simulink model "HIL_simu"  (R2019b)
settings: Solver=VariableStepAuto  StartTime=0.0  StopTime=10.0  RelTol=1e-3
values from neighbouring files (symbols this model uses):
  B = 0.003    [HIL.m]
  b = 7.2e-5    (= 7.2e-05)    [HIL.m]    (also in SIL.m = 4.2697318139e-06)
  C_r = u*Kc/R    (= 0.0265986622074)    [HIL.m]
  Jeq = 0.029*l^2 + J    (= 0.0002543)    [HIL.m]
  K1 = 0.007    [HIL.m]
  K2 = 1    [HIL.m]
  Kc = Ke    (= 0.0241)    [HIL.m]    (also in SIL.m)
  Ke = 24.1e-3    (= 0.0241)    [HIL.m]    (also in SIL.m = 0.024114385317)
  L = 0.42e-3    (= 0.00042)    [HIL.m]    (also in SIL.m)
  R = 2.99    [HIL.m]    (also in SIL.m)
libraries: simulink_extras x2, simulink x1
settings Model: Creator=tclaverie303  LastModifiedBy=tclaverie303

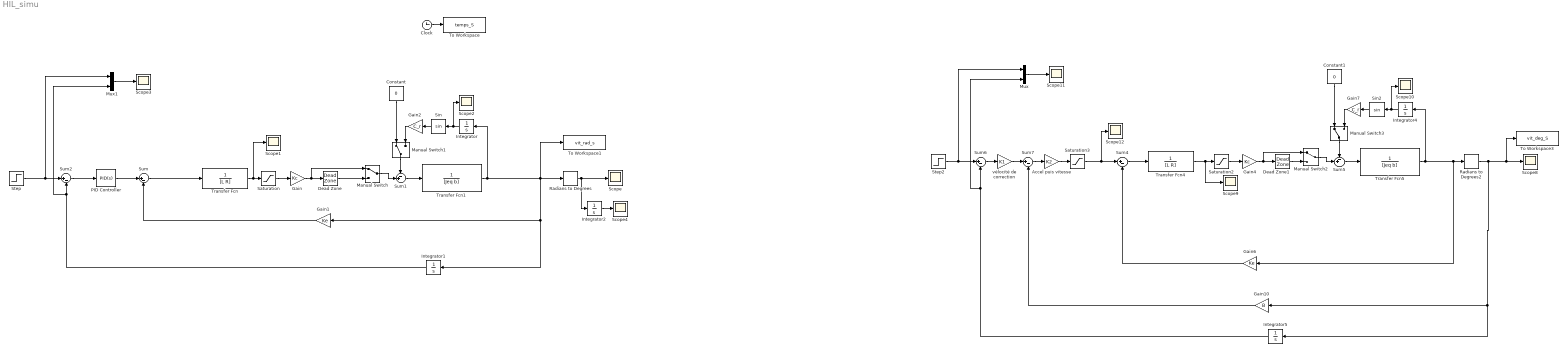
== system HIL_simu ==
  Accel puis vitesse : Gain  Gain=K2
  Clock : Clock
  Constant : Constant  Value=0
  Constant1 : Constant  Value=0
  Dead Zone : DeadZone  SaturateOnIntegerOverflow=on
  Dead Zone1 : DeadZone  SaturateOnIntegerOverflow=on
  Gain : Gain  Gain=Kc
  Gain1 : Gain  Gain=Ke
  Gain10 : Gain  Gain=B
  Gain2 : Gain  Gain=C_r
  Gain4 : Gain  Gain=Kc
  Gain6 : Gain  Gain=Ke
  Gain7 : Gain  Gain=C_r
  Integrator{,1..2,4..5} (5 alike) : Integrator
  Manual Switch{,1..3} (4 alike) : ManualSwitch
  Mux : Mux  Inputs=2
  Mux1 : Mux  Inputs=2
  PID Controller : simulink/Continuous/PID Controller  Controller=PID  Form=Parallel  TimeDomain=Continuous-time  SampleTime=-1  IntegratorMethod=Forward Euler  FilterMethod=Forward Euler  ControllerParametersSource=internal  P=1.5  I=0  D=0.5  UseFilter=on  N=4000  TunerSelectOption=Transfer Function Based (PID Tuner App)  InitialConditionSource=internal  InitialConditionForIntegrator=0  InitialConditionForFilter=0  DifferentiatorICPrevScaledInput=0  ExternalReset=none  TrackingMode=off  Kt=1  LimitOutput=off  UpperSaturationLimit=inf  LowerSaturationLimit=-inf  LinearizeAsGain=on  AntiWindupMode=none  Kb=1  POutMin=[]  POutMax=[]  IOutMin=[]  IOutMax=[]  DOutMin=[]  DOutMax=[]  NOutMin=[]  NOutMax=[]  SumOutMin=[]  SumOutMax=[]  SaturationOutMin=[]  SaturationOutMax=[]  PParamMin=[]  PParamMax=[]  IParamMin=[]  IParamMax=[]  DParamMin=[]  DParamMax=[]  NParamMin=[]  NParamMax=[]  KbParamMin=[]  KbParamMax=[]  KtParamMin=[]  KtParamMax=[]  KbOutMin=[]  KbOutMax=[]  KtOutMin=[]  KtOutMax=[]  IntegratorOutMin=[]  IntegratorOutMax=[]  FilterOutMin=[]  FilterOutMax=[]  SumI1OutMin=[]  SumI1OutMax=[]  SumI2OutMin=[]  SumI2OutMax=[]  SumI3OutMin=[]  SumI3OutMax=[]  SumI4OutMin=[]  SumI4OutMax=[]  SumDOutMin=[]  SumDOutMax=[]  DifferentiatorOutMin=[]  DifferentiatorOutMax=[]  FilterDiffOutCoefMin=[]  FilterDiffOutCoefMax=[]  ReciprocalOutMin=[]  ReciprocalOutMax=[]  SumDenOutMin=[]  SumDenOutMax=[]  SumNumOutMin=[]  SumNumOutMax=[]  DivideOutMin=[]  DivideOutMax=[]  IntegratorContinuousStateAttributes=''  IntegratorStateMustResolveToSignalObject=off  IntegratorRTWStateStorageClass=Auto  FilterContinuousStateAttributes=''  FilterStateMustResolveToSignalObject=off  FilterRTWStateStorageClass=Auto  ParallelPVariant=InternalParameters  IdealPVariant=Disabled  IVariant=InternalParameters  DVariant=InternalParameters  IntegratorVariant=Continuous  SatVariant=Disabled  AWVariant=Passthrough  PCopyVariant=Disabled  TRVariant=Disabled  FdbkBlocksVariant=Forward  IdealPFdbkVariant=Disabled  SatFdbkVariant=Disabled  DerivativeFilterVariant=ContFilter  NVariant=InternalParameters  NCopyVariant=Disabled  FilterICVariant=InternalICsFilter  IntegratorICVariant=InternalICs  ExternalResetVariant=Disabled  TRSumVariant=Passthrough  SumFdbkVariant=Disabled  SumVariant=Sum_PID
  Radians to Degrees : simulink_extras/Transformations/Radians to Degrees
  Radians to Degrees2 : simulink_extras/Transformations/Radians to Degrees
  Saturation : Saturate
  Saturation2 : Saturate
  Saturation3 : Saturate
  Scope{,1..4,8..12} (10 alike) : Scope
  Sin : Trigonometry
  Sin2 : Trigonometry
  Step : Step  After=3.3  SampleTime=0
  Step2 : Step  After=3.3  SampleTime=0
  Sum{,2,4,6..7} (5 alike) : Sum  Inputs=|+-
  Sum1 : Sum  Inputs=-+|
  Sum5 : Sum  Inputs=-+|
  To Workspace : ToWorkspace  VariableName=temps_S  SaveFormat=Timeseries  SampleTime=-1
  To Workspace1 : ToWorkspace  VariableName=vit_rad_s  SaveFormat=Timeseries  SampleTime=-1
  To Workspace3 : ToWorkspace  VariableName=vit_deg_S  SaveFormat=Timeseries  SampleTime=-1
  Transfer Fcn : TransferFcn  Denominator=[L R]
  Transfer Fcn1 : TransferFcn  Denominator=[Jeq b]
  Transfer Fcn4 : TransferFcn  Denominator=[L R]
  Transfer Fcn5 : TransferFcn  Denominator=[Jeq b]
  "vélocité de correction " : Gain  Gain=K1
  wires:
  Sum/1 -> Transfer Fcn/1
  Transfer Fcn/1 -> Scope1/1, Saturation/1
  Saturation/1 -> Gain/1
  Clock/1 -> To Workspace/1
  Gain1/1 -> Sum/2
  Sum1/1 -> Transfer Fcn1/1
  Integrator/1 -> Scope2/1, Sin/1
  Sin/1 -> Gain2/1
  Radians to Degrees/1 -> Integrator2/1, Scope/1
  Gain/1 -> Manual Switch/1, Dead Zone/1
  Dead Zone/1 -> Manual Switch/2
  Manual Switch/1 -> Sum1/2
  Gain2/1 -> Manual Switch1/2
  Manual Switch1/1 -> Sum1/1
  Constant/1 -> Manual Switch1/1
  Sum5/1 -> Transfer Fcn5/1
  Manual Switch2/1 -> Sum5/2
  Dead Zone1/1 -> Manual Switch2/2
  Gain4/1 -> Manual Switch2/1, Dead Zone1/1
  Sin2/1 -> Gain7/1
  Constant1/1 -> Manual Switch3/1
  Gain7/1 -> Manual Switch3/2
  Manual Switch3/1 -> Sum5/1
  Integrator4/1 -> Scope10/1, Sin2/1
  Gain6/1 -> Sum4/2
  Radians to Degrees2/1 -> Integrator5/1, Gain10/1, To Workspace3/1, Scope8/1
  Transfer Fcn5/1 -> Integrator4/1, Radians to Degrees2/1, Gain6/1
  Transfer Fcn4/1 -> Scope9/1, Saturation2/1
  Sum4/1 -> Transfer Fcn4/1
  Saturation2/1 -> Gain4/1
  Step2/1 -> Mux/1, Sum6/1
  Sum6/1 -> "vélocité de correction "/1
  "vélocité de correction "/1 -> Sum7/1
  Sum7/1 -> Accel puis vitesse/1
  Accel puis vitesse/1 -> Saturation3/1
  Saturation3/1 -> Scope12/1, Sum4/1
  Gain10/1 -> Sum7/2
  Integrator5/1 -> Mux/2, Sum6/2
  Mux/1 -> Scope11/1
  PID Controller/1 -> Sum/1
  Sum2/1 -> PID Controller/1
  Transfer Fcn1/1 -> Integrator/1, Radians to Degrees/1, To Workspace1/1, Integrator1/1, Gain1/1
  Mux1/1 -> Scope3/1
  Step/1 -> Mux1/1, Sum2/1
  Integrator1/1 -> Mux1/2, Sum2/2
  Integrator2/1 -> Scope4/1
